simulink model "noAppliMdl"  (Simulink 7.8)
settings: Solver=ode45  StartTime=0  StopTime=170  RelTol=1e-3
libraries: ApplFwS1v1_LIB x2, simulink x1
settings Model: Creator=z0035ypc  LastModifiedBy=z003019m

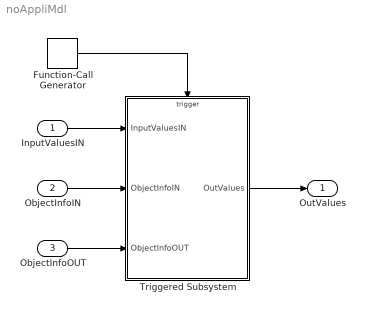
== system noAppliMdl ==
  InputValuesIN : Inport  PortDimensions=3  Interpolate=off
  ObjectInfoIN : Inport  Port=2  PortDimensions=3  Interpolate=off
  ObjectInfoOUT : Inport  Port=3  PortDimensions=3  Interpolate=off
  Function-Call Generator : simulink/Ports & Subsystems/Function-Call Generator  sample_time=0.2  numberOfIterations=1
  Triggered Subsystem : Subsystem  TreatAsAtomicUnit=on
  OutValues : Outport
  wires:
  InputValuesIN/1 -> Triggered Subsystem/1(InputValuesIN)
  ObjectInfoIN/1 -> Triggered Subsystem/2(ObjectInfoIN)
  ObjectInfoOUT/1 -> Triggered Subsystem/3(ObjectInfoOUT)
  Function-Call Generator/1 -> Triggered Subsystem/Trigger
  Triggered Subsystem/1(OutValues) -> OutValues/1

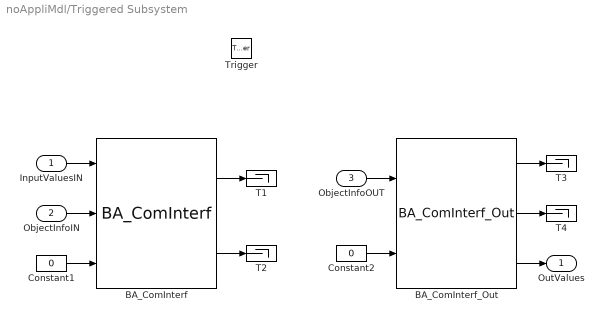
== system noAppliMdl/Triggered Subsystem ==
  InputValuesIN : Inport
  ObjectInfoIN : Inport  Port=2
  ObjectInfoOUT : Inport  Port=3
  Trigger : TriggerPort  TriggerType=function-call
  BA_ComInterf : ApplFwS1v1_LIB/XFB/BA_ComInterf  DeviceId=4194303  ObjectId=4194303
  BA_ComInterf_Out : ApplFwS1v1_LIB/XFB/BA_ComInterf_Out  DeviceId=4194303  ObjectId=333
  Constant1 : Constant  Value=0
  Constant2 : Constant  Value=0
  T{1..4} (4 alike) : Terminator
  OutValues : Outport
  wires:
  InputValuesIN/1 -> BA_ComInterf/1
  ObjectInfoIN/1 -> BA_ComInterf/2
  Constant1/1 -> BA_ComInterf/3
  ObjectInfoOUT/1 -> BA_ComInterf_Out/1
  Constant2/1 -> BA_ComInterf_Out/2
  BA_ComInterf/1 -> T1/1
  BA_ComInterf/2 -> T2/1
  BA_ComInterf_Out/1 -> T3/1
  BA_ComInterf_Out/2 -> T4/1
  BA_ComInterf_Out/3 -> OutValues/1
